simulink model "test_pwm_aux_out_01"  (Simulink 8.8)
settings: Solver=FixedStepDiscrete  StartTime=0.0  StopTime=10.0  FixedStep=0.01  RelTol=1e-3  EnableMultiTasking=on
InitFcn:
  | px4_ap1_mdl_callback('check_model');
libraries: px4_ap1_pwm_aux_out_lib x1, px4_ap1_px4setup_lib x1
settings Model: Creator=Privat  LastModifiedBy=Privat
settings OptimizationCC: ExpressionDepthLimit=2147483647  InitFltsAndDblsToZero=on  LifeSpan=1
settings DebuggingCC: SolverPrmCheckMsg=warning  InheritedTsInSrcMsg=none  StrictBusMsg=Warning
settings RTWCC: SystemTargetFile=px4_ap1.tlc  GenCodeOnly=on  GenerateMakefile=off
settings CodeAppCC: IgnoreCustomStorageClasses=off  CustomSymbolStrType=$N$R$M  InternalIdentifier=Classic
settings STFCustomTargetCC: ModelReferenceCompliant=off  IncludeMdlTerminateFcn=off  CombineOutputUpdateFcns=on  ERTCustomFileBanners=on  SupportContinuousTime=off  SupportNonInlinedSFcns=off  RemoveResetFunc=on  MATLABClassNameForMDSCustomization=Simulink.SoftwareTarget.ERTCustomization  CPPClassGenCompliant=on  GRTInterface=off  SystemTargetFile=px4_ap1.tlc
settings ERTTargetCC: MultiwordLength=2048  ModelReferenceCompliant=off  ParMdlRefBuildCompliant=off  CompOptLevelCompliant=off  ConcurrentExecutionCompliant=off  IncludeMdlTerminateFcn=off  ERTFirstTimeCompliant=off  ModelStepFunctionPrototypeControlCompliant=off  UseToolchainInfoCompliant=off  ERTSrcFileBannerTemplate=px4_ap1_code_template.cgt  ERTHdrFileBannerTemplate=px4_ap1_code_template.cgt  ERTDataSrcFileTemplate=px4_ap1_code_template.cgt  ERTDataHdrFileTemplate=px4_ap1_code_template.cgt  ERTCustomFileTemplate=px4_ap1_main.tlc  ConvertIfToSwitch=off  SuppressUnreachableDefaultCases=off

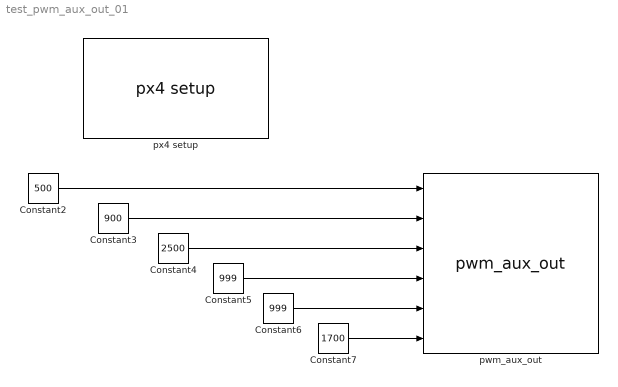
== system test_pwm_aux_out_01 ==
  Constant2 : Constant  Value=500  OutDataTypeStr=uint16
  Constant3 : Constant  Value=900  OutDataTypeStr=uint16
  Constant4 : Constant  Value=2500  OutDataTypeStr=uint16
  Constant5 : Constant  Value=999  OutDataTypeStr=uint16
  Constant6 : Constant  Value=999  OutDataTypeStr=uint16
  Constant7 : Constant  Value=1700  OutDataTypeStr=uint16
  pwm_aux_out : px4_ap1_pwm_aux_out_lib/pwm_aux_out  Description=Setup for PX4 native software  aux1=on  aux2=on  aux3=on  aux4=on  aux5=on  aux6=on  pwm_1_4=19  pwm_5_6=401
  px4 setup : px4_ap1_px4setup_lib/px4 setup  SampleTimeValue=0.01  cbBuild=on  cbUpload=off  cbPort=COM3  cpuLoad=off  debugmode=on
  wires:
  Constant2/1 -> pwm_aux_out/1
  Constant3/1 -> pwm_aux_out/2
  Constant4/1 -> pwm_aux_out/3
  Constant5/1 -> pwm_aux_out/4
  Constant6/1 -> pwm_aux_out/5
  Constant7/1 -> pwm_aux_out/6
